simulink model "normal_forces"  (R2015a)
settings: Solver=ode45  StartTime=0.0  StopTime=10.0  RelTol=1e-3
undefined symbols (not defined in the file): h, l, l_f, l_r, l_w, m
settings Model: Creator=BML  LastModifiedBy=BML

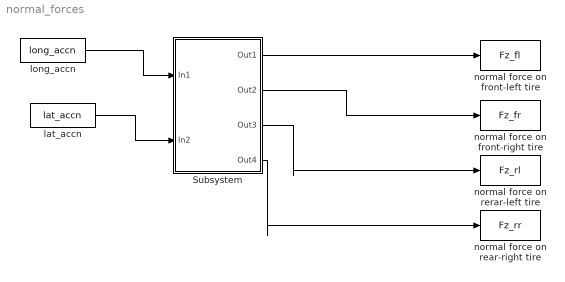
== system normal_forces ==
  Subsystem : Subsystem
  lat_accn : FromWorkspace  VariableName=lat_accn  SampleTime=0
  long_accn : FromWorkspace  VariableName=long_accn  SampleTime=0
  normal force on front-left tire : ToWorkspace  VariableName=Fz_fl  SaveFormat=Timeseries  SampleTime=-1
  normal force on front-right tire : ToWorkspace  VariableName=Fz_fr  SaveFormat=Timeseries  SampleTime=-1
  normal force on rear-right tire : ToWorkspace  VariableName=Fz_rr  SaveFormat=Timeseries  SampleTime=-1
  normal force on rerar-left tire : ToWorkspace  VariableName=Fz_rl  SaveFormat=Timeseries  SampleTime=-1
  wires:
  long_accn/1 -> Subsystem/1(In1)
  lat_accn/1 -> Subsystem/2(In2)
  Subsystem/1(Out1) -> normal force on front-left tire/1
  Subsystem/2(Out2) -> normal force on front-right tire/1
  Subsystem/3(Out3) -> normal force on rerar-left tire/1
  Subsystem/4(Out4) -> normal force on rear-right tire/1

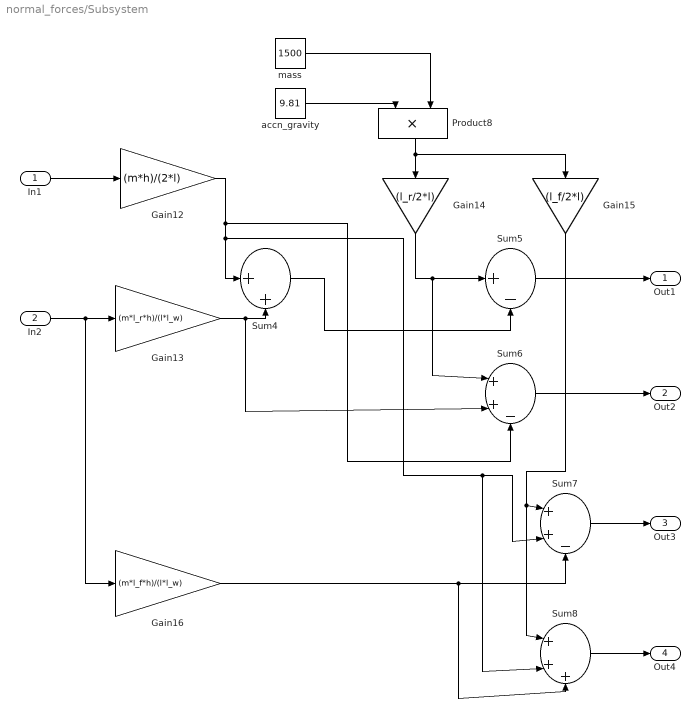
== system normal_forces/Subsystem ==
  In1 : Inport
  In2 : Inport  Port=2
  Gain12 : Gain  Gain=(m*h)/(2*l)
  Gain13 : Gain  Gain=(m*l_r*h)/(l*l_w)
  Gain14 : Gain  Gain=(l_r/2*l)
  Gain15 : Gain  Gain=(l_f/2*l)
  Gain16 : Gain  Gain=(m*l_f*h)/(l*l_w)
  Product8 : Product
  Sum4 : Sum  Inputs=|++
  Sum5 : Sum  Inputs=|+-
  Sum6 : Sum  Inputs=|++-
  Sum7 : Sum  Inputs=|++-
  Sum8 : Sum  Inputs=|+++
  "accn_gravity " : Constant  Value=9.81
  mass : Constant  Value=1500
  Out1 : Outport
  Out2 : Outport  Port=2
  Out3 : Outport  Port=3
  Out4 : Outport  Port=4
  wires:
  Gain12/1 -> Sum4/1, Sum8/2, Sum7/2, Sum6/3
  Gain15/1 -> Sum8/1, Sum7/1
  Gain16/1 -> Sum8/3, Sum7/3
  Sum7/1 -> Out3/1
  In2/1 -> Gain16/1, Gain13/1
  Gain13/1 -> Sum6/2, Sum4/2
  Sum5/1 -> Out1/1
  Sum6/1 -> Out2/1
  Sum4/1 -> Sum5/2
  In1/1 -> Gain12/1
  mass/1 -> Product8/2
  Gain14/1 -> Sum5/1, Sum6/1
  Sum8/1 -> Out4/1
  Product8/1 -> Gain15/1, Gain14/1
  "accn_gravity "/1 -> Product8/1
